simulink model "Lab2_4"  (Simulink 7.3)
settings: Solver=ode45  StartTime=0.0  StopTime=10.0  RelTol=1e-3
libraries: simulink x2
settings Model: Creator=Seva  LastModifiedBy=Seva

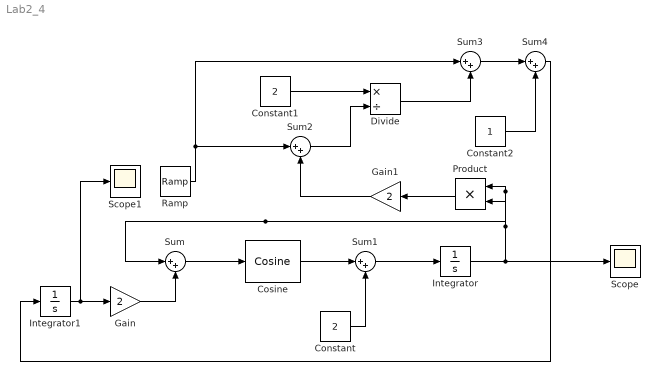
== system Lab2_4 ==
  Constant : Constant  Value=2  OutDataType=fixdt(1, 16)  OutScaling=2^0
  Constant1 : Constant  Value=2  OutDataType=fixdt(1, 16)  OutScaling=2^0
  Constant2 : Constant  OutDataType=fixdt(1, 16)  OutScaling=2^0
  Cosine : simulink/Lookup Tables/Cosine  SystemSampleTime=-1  Formula=cos(2*pi*u)  NumDataPoints=(2^5)+1  OutputWordLength=16
  Divide : Product  Inputs=*/  OutDataType=fixdt(1, 16)  OutScaling=2^-10
  Gain : Gain  Gain=2  ParameterDataType=fixdt(1, 16)  ParameterScaling=2^0  OutDataType=fixdt(1, 16)  OutScaling=2^0
  Gain1 : Gain  Gain=2  ParameterDataType=fixdt(1, 16)  ParameterScaling=2^0  OutDataType=fixdt(1, 16)  OutScaling=2^0
  Integrator : Integrator  InitialCondition=1
  Integrator1 : Integrator  InitialCondition=0.005
  Product : Product  OutDataType=fixdt(1, 16)  OutScaling=2^0  RndMeth=Zero
  Ramp : simulink/Sources/Ramp  SystemSampleTime=-1  slope=1  start=0  X0=0
  Scope : Scope
  Scope1 : Scope
  Sum{,1..4} (5 alike) : Sum  Inputs=|++  OutDataType=fixdt(1, 16)  OutScaling=2^0
  wires:
  Gain/1 -> Sum/2
  Sum/1 -> Cosine/1
  Cosine/1 -> Sum1/1
  Constant/1 -> Sum1/2
  Sum1/1 -> Integrator/1
  Integrator/1 -> Product/1, Product/2, Sum/1, Scope/1
  Ramp/1 -> Sum2/1, Sum3/1
  Product/1 -> Gain1/1
  Gain1/1 -> Sum2/2
  Constant1/1 -> Divide/1
  Sum2/1 -> Divide/2
  Divide/1 -> Sum3/2
  Sum3/1 -> Sum4/1
  Constant2/1 -> Sum4/2
  Integrator1/1 -> Gain/1, Scope1/1
  Sum4/1 -> Integrator1/1
